simulink model "sampleModel1891"  (R2023a)
settings: Solver=VariableStepAuto  StartTime=0.0  StopTime=10.0  RelTol=1e-3
libraries: hdlsllib x9, simulink x1
settings Model: Creator=user1  LastModifiedBy=user1

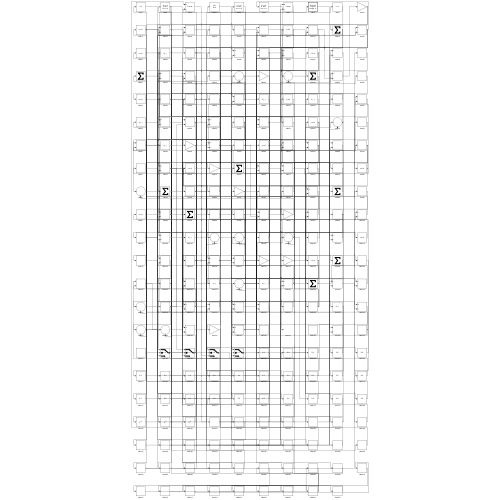
[thumbnail: Simulink's stored preview of the top-level diagram]
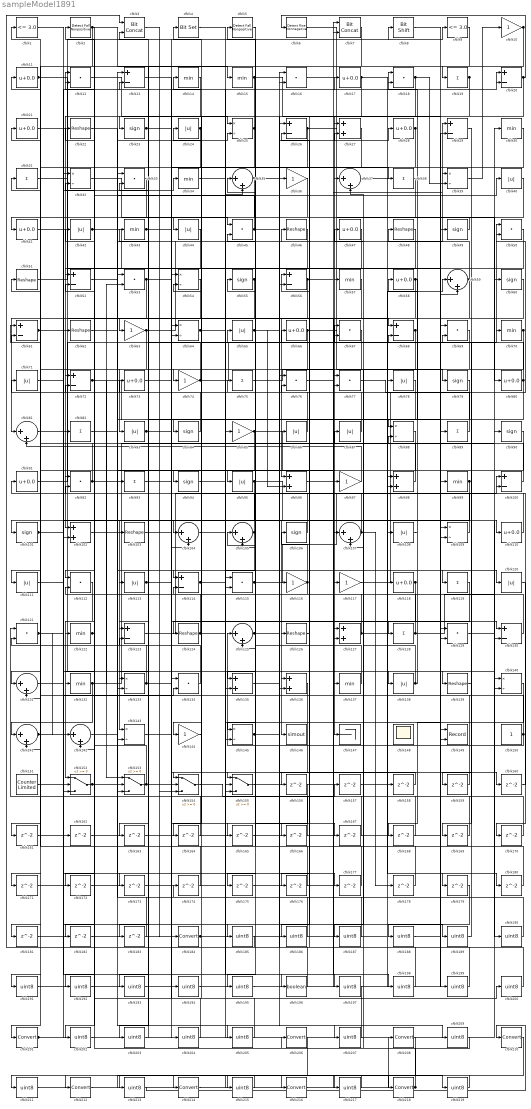
== system sampleModel1891 ==
  cfblk1 : hdlsllib/Logic and Bit Operations/Compare To Constant  relop=<=  const=3.0  OutDataTypeStr=boolean
  cfblk{10,36,63,74,85,97,116..117,144} (9 alike) : Gain
  cfblk{13,20,26,29,52,56,61,68,72,100,114,123,130} (13 alike) : Sum  Inputs=+-
  cfblk{23,49,55,60,79,84,90,94,101,106} (10 alike) : Signum
  cfblk{27,96,98,102,127,135..136} (7 alike) : Sum
  cfblk{22,46,48,51,62,103,124,126,139} (9 alike) : Reshape
  cfblk{35,37,59,81,104..105,107,125,131,141..142} (11 alike) : Sum  Inputs=|++
  cfblk{24,40,42,44,65,71,78,83,86..87,95,108,111,113,120,138} (16 alike) : Abs  SaturateOnIntegerOverflow=off
  cfblk{25,32,39,54,64,88,109,133,140,143,145} (11 alike) : Product  Inputs=*/  RndMeth=Zero  SaturateOnIntegerOverflow=on
  cfblk{11,17,21,28,41,47,58,66,73,80,91,110,118} (13 alike) : Bias  Bias=0.0  SaturateOnIntegerOverflow=off
  cfblk{12,16,18,33,45,50,53,67,69,76..77,92,112,115,121,129,134} (17 alike) : DotProduct  OutDataTypeStr=Inherit: Inherit via internal rule
  cfblk{19,31,38,75,82,89,93,119,128} (9 alike) : Sum  Inputs=+
  cfblk{14..15,30,34,43,57,70,99,122,132,137} (11 alike) : MinMax
  cfblk146 : ToWorkspace  VariableName=simout  SaveFormat=Timeseries  SampleTime=-1
  cfblk147 : Terminator
  cfblk148 : Scope
      settings: Floating=on
  cfblk149 : Record  FileSettingsInternal="{\"entries\":[{\"content\":{\"excelSettings\":{\"content\":{},\"type\":\"Streamout.ExcelSettings\"}},\"type\":\"Streamout.FileSettingStorage\",\"uuid\":\"\"}],\"packageUris\":[\"http:\\/\\/schema.mathworks.com\\/mf0\\/streamout_blocks\\/R2020a\"],\"version\":\"1.0\"}"  Layout=[1 1]  SignalsInternal="{\"entries\":[{\"content\":{\"signals\":[{\"content\":{\"blockPath\":[],\"dimensions\":[1],\"domain\":\"\",\"lineColor\":\"#a2142f\",\"plots\":[1],\"port\":1,\"signalID\":4842,\"signalName\":\"XY Graph:1\"},\"type\":\"RecordBlkView.Signal\",\"uuid\":\"\"},{\"content\":{\"blockPath\":[],\"dimensions\":[1],\"domain\":\"\",\"lineColor\":\"#139fff\",\"plots\":[1],\"port\":2,\"signalID\":4845,\"signalName\":\"XY Graph:2\"},\"type\":\"RecordBlkView.Signal\",\"uuid\":\"\"}]},\"type\":\"RecordBlkView.InputSignals\",\"uuid\":\"\"}],\"packageUris\":[\"http:\\/\\/schema.mathworks.com\\/mf0\\/streamout_blocks\\/R2020a\"],\"version\":\"1.0\"}"  VisualizationBindings="{\"xyplotplugin\":{\"info\":[{\"series\":[{\"bindingParametersList\":[{\"parameter\":\"X-Axis\",\"signalID\":4842,\"signalName\":\"XY Graph:1\"},{\"parameter\":\"Y-Axis\",\"signalID\":4845,\"signalName\":\"XY Graph:2\"}],\"seriesID\":37107}],\"subplotID\":1}]}}"  CompatibilityTag=XY  st=-1
  cfblk150 : Constant  SampleTime=-1
  cfblk151 : hdlsllib/Sources/Counter Limited  uplimit=7  tsamp=-1
  cfblk{152..155} (4 alike) : Switch  SaturateOnIntegerOverflow=off  InputSameDT=off
  cfblk{156..183} (28 alike) : Delay  SampleTime=1
  cfblk{184,201,206,208,210,212,214,216,218} (9 alike) : DataTypeConversion  SaturateOnIntegerOverflow=off  RndMeth=Floor
  cfblk{185..195,197..200,202..205,207,209,211,213,215,217,219} (26 alike) : DataTypeConversion  OutDataTypeStr=uint8  SaturateOnIntegerOverflow=off  RndMeth=Floor
  cfblk196 : DataTypeConversion  OutDataTypeStr=boolean  SaturateOnIntegerOverflow=off  RndMeth=Floor
  cfblk2 : hdlsllib/Logic and Bit Operations/Detect Fall Nonpositive  vinit=0  OutDataTypeStr=boolean
  cfblk3 : hdlsllib/Logic and Bit Operations/Bit Concat  numInputs=2
  cfblk4 : simulink/Logic and Bit Operations/Bit Set  iBit=0
      settings: LibrarySourceBlock=|
      | hdlsllib/Logic and Bit
      | Operations/Bit Set
  cfblk5 : hdlsllib/Logic and Bit Operations/Detect Fall Nonpositive  vinit=0  OutDataTypeStr=boolean
  cfblk6 : hdlsllib/Logic and Bit Operations/Detect Rise Nonnegative  vinit=0  OutDataTypeStr=boolean
  cfblk7 : hdlsllib/Logic and Bit Operations/Bit Concat  numInputs=2
  cfblk8 : hdlsllib/Logic and Bit Operations/Bit Shift  mode=Shift Left Logical  N=0
  cfblk9 : hdlsllib/Logic and Bit Operations/Compare To Constant  relop=<=  const=3.0  OutDataTypeStr=boolean
  wires:
  cfblk17/1 -> cfblk147/1, cfblk37/1, cfblk180/1
  cfblk58/1 -> cfblk96/1, cfblk88/1
  cfblk60/1 -> cfblk201/1
  cfblk112/1 -> cfblk152/1
  cfblk90/1 -> cfblk94/1
  cfblk130/1 -> cfblk35/1
  cfblk75/1 -> cfblk77/1
  cfblk150/1 -> cfblk125/1, cfblk71/1
  cfblk77/1 -> cfblk50/1
  cfblk128/1 -> cfblk105/1, cfblk90/1
  cfblk153/1 -> cfblk91/1, cfblk70/1
  cfblk41/1 -> cfblk139/1
  cfblk88/1 -> cfblk101/1
  cfblk25/1 -> cfblk23/1, cfblk124/1
  cfblk18/1 -> cfblk102/1, cfblk39/2
  cfblk61/1 -> cfblk143/1, cfblk13/2
  cfblk91/1 -> cfblk65/1
  cfblk49/1 -> cfblk44/1
  cfblk99/1 -> cfblk146/1, cfblk161/1
  cfblk63/1 -> cfblk29/1, cfblk153/3
  cfblk138/1 -> cfblk48/1, cfblk67/2, cfblk37/2
  cfblk6/1 -> cfblk79/1
  cfblk34/1 -> cfblk126/1
  cfblk40/1 -> cfblk111/1
  cfblk116/1 -> cfblk106/1, cfblk114/2
  cfblk68/1 -> cfblk83/1, cfblk191/1
  cfblk134/1 -> cfblk11/1
  cfblk105/1 -> cfblk14/1, cfblk133/2
  cfblk12/1 -> cfblk25/1
  cfblk137/1 -> cfblk55/1
  cfblk123/1 -> cfblk36/1
  cfblk132/1 -> cfblk30/1, cfblk53/2, cfblk181/1
  cfblk82/1 -> cfblk97/1
  cfblk117/1 -> cfblk49/1
  cfblk64/1 -> cfblk128/1, cfblk149/2
  cfblk94/1 -> cfblk35/2
  cfblk115/1 -> cfblk29/2, cfblk160/1
  cfblk24/1 -> cfblk114/1, cfblk192/1
  cfblk155/1 -> cfblk98/1
  cfblk81/1 -> cfblk143/2
  cfblk55/1 -> cfblk81/1, cfblk64/2
  cfblk50/1 -> cfblk82/1
  cfblk74/1 -> cfblk50/2, cfblk43/1
  cfblk121/1 -> cfblk62/1, cfblk142/1
  cfblk32/1 -> cfblk45/1
  cfblk113/1 -> cfblk66/1, cfblk88/2
  cfblk39/1 -> cfblk10/1
  cfblk3/1 -> cfblk184/1
  cfblk51/1 -> cfblk8/1
  cfblk9/1 -> cfblk19/1
  cfblk59/1 -> cfblk123/1, cfblk18/1
  cfblk20/1 -> cfblk6/1, cfblk56/2, cfblk175/1, cfblk176/1
  cfblk21/1 -> cfblk57/1
  cfblk86/1 -> cfblk75/1
  cfblk151/1 -> cfblk34/1
  cfblk114/1 -> cfblk85/1, cfblk17/1
  cfblk80/1 -> cfblk145/1, cfblk24/1
  cfblk31/1 -> cfblk77/2
  cfblk127/1 -> cfblk59/1, cfblk73/1
  cfblk85/1 -> cfblk117/1, cfblk142/2
  cfblk46/1 -> cfblk132/1
  cfblk33/1 -> cfblk122/1
  cfblk97/1 -> cfblk81/2
  cfblk35/1 -> cfblk41/1, cfblk120/1
  cfblk101/1 -> cfblk20/1, cfblk177/1
  cfblk53/1 -> cfblk72/1, cfblk130/1
  cfblk118/1 -> cfblk154/1, cfblk136/2
  cfblk141/1 -> cfblk173/1, cfblk196/1
  cfblk131/1 -> cfblk134/2
  cfblk124/1 -> cfblk92/2, cfblk166/1
  cfblk66/1 -> cfblk109/1, cfblk153/2
  cfblk57/1 -> cfblk102/2
  cfblk104/1 -> cfblk119/1
  cfblk27/1 -> cfblk52/1
  cfblk15/1 -> cfblk89/1, cfblk92/1
  cfblk152/1 -> cfblk53/1, cfblk46/1
  cfblk133/1 -> cfblk9/1, cfblk121/2
  cfblk23/1 -> cfblk154/3, cfblk165/1
  cfblk38/1 -> cfblk135/1
  cfblk145/1 -> cfblk100/1, cfblk20/2, cfblk125/2
  cfblk2/1 -> cfblk152/3, cfblk112/1, cfblk15/1
  cfblk42/1 -> cfblk149/1, cfblk108/1
  cfblk125/1 -> cfblk87/1, cfblk68/2, cfblk27/2
  cfblk142/1 -> cfblk25/2
  cfblk19/1 -> cfblk144/1, cfblk27/1
  cfblk79/1 -> cfblk133/1
  cfblk72/1 -> cfblk99/1, cfblk116/1, cfblk153/1
  cfblk106/1 -> cfblk52/2
  cfblk43/1 -> cfblk68/1, cfblk95/1
  cfblk109/1 -> cfblk67/1
  cfblk102/1 -> cfblk103/1
  cfblk122/1 -> cfblk12/2, cfblk182/1
  cfblk10/1 -> cfblk171/1, cfblk172/1
  cfblk126/1 -> cfblk56/1
  cfblk70/1 -> cfblk141/1, cfblk107/2
  cfblk30/1 -> cfblk86/1
  cfblk92/1 -> cfblk21/1, cfblk140/2
  cfblk65/1 -> cfblk137/1, cfblk96/2
  cfblk71/1 -> cfblk110/1
  cfblk67/1 -> cfblk115/2
  cfblk98/1 -> cfblk61/2
  cfblk110/1 -> cfblk51/1
  cfblk47/1 -> cfblk63/1
  cfblk52/1 -> cfblk40/1
  cfblk13/1 -> cfblk38/1
  cfblk96/1 -> cfblk39/1
  cfblk119/1 -> cfblk155/3
  cfblk62/1 -> cfblk84/1
  cfblk5/1 -> cfblk105/2
  cfblk56/1 -> cfblk141/2, cfblk18/2
  cfblk89/1 -> cfblk5/1
  cfblk87/1 -> cfblk31/1
  cfblk84/1 -> cfblk12/1
  cfblk16/1 -> cfblk80/1
  cfblk100/1 -> cfblk26/2
  cfblk44/1 -> cfblk113/1
  cfblk108/1 -> cfblk58/1
  cfblk136/1 -> cfblk154/2
  cfblk11/1 -> cfblk93/1, cfblk138/1
  cfblk107/1 -> cfblk42/1, cfblk178/1
  cfblk26/1 -> cfblk104/1, cfblk118/1
  cfblk93/1 -> cfblk136/1
  cfblk83/1 -> cfblk109/2, cfblk130/2
  cfblk45/1 -> cfblk2/1, cfblk207/1
  cfblk135/1 -> cfblk28/1
  cfblk28/1 -> cfblk131/1, cfblk74/1
  cfblk95/1 -> cfblk140/1, cfblk183/1
  cfblk78/1 -> cfblk156/1
  cfblk154/1 -> cfblk157/1
  cfblk157/1 -> cfblk98/2
  cfblk158/1 -> cfblk155/1
  cfblk29/1 -> cfblk159/1
  cfblk159/1 -> cfblk61/1
  cfblk160/1 -> cfblk100/2
  cfblk161/1 -> cfblk16/2
  cfblk111/1 -> cfblk162/1
  cfblk14/1 -> cfblk163/1
  cfblk163/1 -> cfblk135/2
  cfblk144/1 -> cfblk164/1
  cfblk164/1 -> cfblk152/2
  cfblk165/1 -> cfblk59/2
  cfblk166/1 -> cfblk26/1
  cfblk103/1 -> cfblk167/1
  cfblk167/1 -> cfblk72/2
  cfblk140/1 -> cfblk168/1
  cfblk168/1 -> cfblk121/1
  cfblk139/1 -> cfblk169/1
  cfblk169/1 -> cfblk127/1
  cfblk120/1 -> cfblk170/1
  cfblk170/1 -> cfblk64/1
  cfblk171/1 -> cfblk155/2
  cfblk172/1 -> cfblk145/2
  cfblk173/1 -> cfblk123/2
  cfblk174/1 -> cfblk134/1
  cfblk175/1 -> cfblk107/1
  cfblk176/1 -> cfblk131/2
  cfblk177/1 -> cfblk45/2
  cfblk178/1 -> cfblk32/2
  cfblk37/1 -> cfblk179/1
  cfblk180/1 -> cfblk1/1
  cfblk181/1 -> cfblk104/2
  cfblk183/1 -> cfblk13/1
  cfblk184/1 -> cfblk158/1, cfblk127/2
  cfblk162/1 -> cfblk185/1
  cfblk185/1 -> cfblk3/1
  cfblk48/1 -> cfblk186/1
  cfblk186/1 -> cfblk3/2
  cfblk69/1 -> cfblk187/1
  cfblk187/1 -> cfblk16/1
  cfblk179/1 -> cfblk188/1
  cfblk188/1 -> cfblk69/1
  cfblk1/1 -> cfblk189/1
  cfblk189/1 -> cfblk69/2
  cfblk129/1 -> cfblk190/1
  cfblk190/1 -> cfblk33/1
  cfblk191/1 -> cfblk129/1
  cfblk192/1 -> cfblk129/2
  cfblk7/1 -> cfblk193/1
  cfblk193/1 -> cfblk78/1
  cfblk143/1 -> cfblk194/1
  cfblk194/1 -> cfblk7/1
  cfblk156/1 -> cfblk195/1
  cfblk195/1 -> cfblk7/2
  cfblk196/1 -> cfblk4/1
  cfblk4/1 -> cfblk197/1
  cfblk76/1 -> cfblk198/1
  cfblk198/1 -> cfblk174/1
  cfblk8/1 -> cfblk199/1
  cfblk199/1 -> cfblk76/1
  cfblk197/1 -> cfblk200/1
  cfblk200/1 -> cfblk76/2
  cfblk201/1 -> cfblk32/1, cfblk115/1
  cfblk36/1 -> cfblk202/1
  cfblk202/1 -> cfblk60/1
  cfblk54/1 -> cfblk203/1
  cfblk203/1 -> cfblk33/2
  cfblk73/1 -> cfblk204/1
  cfblk204/1 -> cfblk54/1
  cfblk182/1 -> cfblk205/1
  cfblk205/1 -> cfblk54/2
  cfblk207/1 -> cfblk22/1
  cfblk22/1 -> cfblk209/1
  cfblk209/1 -> cfblk206/1
  cfblk206/1 -> cfblk211/1
  cfblk211/1 -> cfblk208/1
  cfblk208/1 -> cfblk213/1
  cfblk213/1 -> cfblk210/1
  cfblk210/1 -> cfblk215/1
  cfblk215/1 -> cfblk212/1
  cfblk216/1 -> cfblk218/1
  cfblk212/1 -> cfblk217/1
  cfblk217/1 -> cfblk214/1
  cfblk218/1 -> cfblk112/2, cfblk47/1
  cfblk214/1 -> cfblk219/1
  cfblk219/1 -> cfblk216/1
